simulink model "SIMU_OPAM_CHIDO"  (R2025b)
settings: Solver=ode23t  StartTime=0.0  StopTime=0.02  RelTol=1e-3
values from neighbouring files (symbols this model uses):
  a = (R1*R2*R3*C1*C2)/(R3+R4)    (= 4e-09)    [Circuito.m]    (also in Parametros.m)
  b = (R1*R3*C1 + R2*R3*C1 - R1*R4*C2)/(R3+R4)    (= 2e-05)    [Circuito.m]    (also in Parametros.m)
  c = R3/(R3+R4)    (= 0.4)    [Circuito.m]    (also in Parametros.m)
settings Model: Creator=dpaul  LastModifiedBy=dpaul

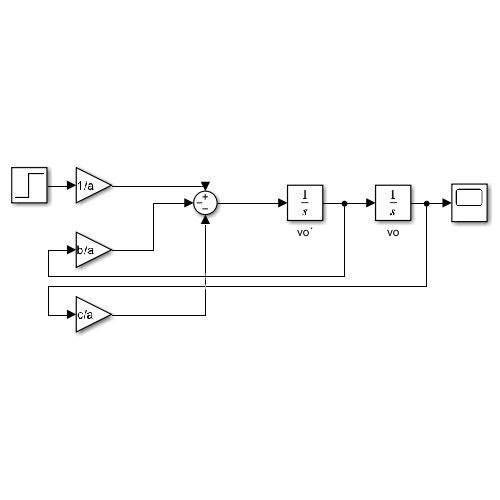
[thumbnail: Simulink's stored preview of the top-level diagram]
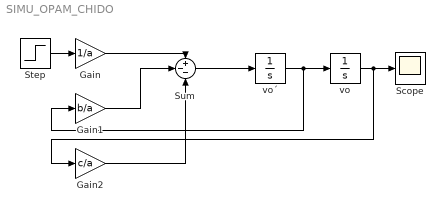
== system SIMU_OPAM_CHIDO ==
  Gain : Gain  Gain=1/a
  Gain1 : Gain  Gain=b/a
  Gain2 : Gain  Gain=c/a
  Scope : Scope
      settings: TimeSpan=0.01  ActiveDisplayYMinimum=-0.45136683278345213  ActiveDisplayYMaximum=4.06230149505107
  Step : Step  Time=0  SampleTime=0
  Sum : Sum  Inputs=+--
  vo : Integrator
  vo´ : Integrator
  wires:
  vo/1 -> Scope/1, Gain2/1
  vo´/1 -> Gain1/1, vo/1
  Gain/1 -> Sum/1
  Gain1/1 -> Sum/2
  Sum/1 -> vo´/1
  Gain2/1 -> Sum/3
  Step/1 -> Gain/1
